simulink model "ble"  (R2020a)
settings: Solver=FixedStepAuto  StartTime=0.0  StopTime=10.0  RelTol=1e-3
undefined symbols (not defined in the file): B3, B7, BLE_Receive, BLE_Send, data, F0, untitled
libraries: androidcommunicationlib x2, androiduilib x2
settings Model: Creator=luisi  LastModifiedBy=luisi
settings OptimizationCC: EnhancedBackFolding=on  PassReuseOutputArgsAs=Individual arguments  ZeroExternalMemoryAtStartup=off  ZeroInternalMemoryAtStartup=off  MaxStackSize=64  OptimizeBlockOrder=speed  DifferentSizesBufferReuse=on  OptimizationCustomize=off  EfficientTunableParamExpr=on
settings DebuggingCC: ParameterTunabilityLossMsg=error
settings HardwareCC: ProdBitPerPointer=32  ProdBitPerSizeT=32  ProdBitPerPtrDiffT=32  ProdLargestAtomicInteger=Long  ProdLargestAtomicFloat=Double  ProdWordSize=32  ProdHWDeviceType=ARM Compatible->ARM Cortex
settings SFSimCC: MATLABDynamicMemAlloc=off
settings RTWCC: SystemTargetFile=ert.tlc  HardwareBoard=Android Device  TemplateMakefile=ert_default_tmf  RTWVerbose=off  Toolchain=Android SDK/NDK Tools
settings CodeAppCC: ForceParamTrailComments=on  IgnoreCustomStorageClasses=off  OperatorAnnotations=on  SimulinkDataObjDesc=on  SFDataObjDesc=on  InsertBlockDesc=on
settings ERTTargetCC: ExtModeMexArgs='192.168.0.149'

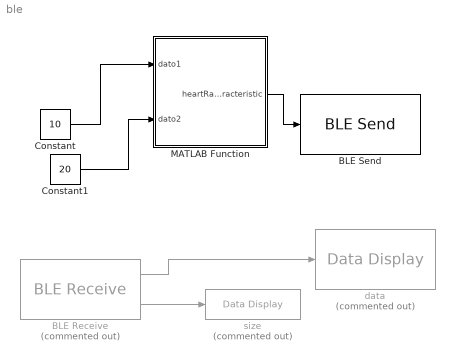
== system ble ==
  BLE Receive : androidcommunicationlib/BLE Receive  Commented=on  DeviceMode=Central (Client)  BluetoothAddress=44:B7:F0:20:80:B3  CharUUID=00002a01-0000-1000-8000-00805f9b34fb  ServiceUUID=00001800-0000-1000-8000-00805f9b34fb  device=RedmiLuisa  character=Generic Access\Appearance  CustomService=off  ServiceName=Heart Rate  CharacteristicName="Heart Rate  Measurement"  CustomServiceUUID=<Enter Service UUID>  CustomCharUUID=<Enter Characteristic UUID>  DataSize=2  SampleTime=0.1  charseruuid=00001801-0000-1000-8000-00805f9b34fb\00002a05-0000-1000-8000-00805f9b34fb  seruuid=00001810-0000-1000-8000-00805f9b34fb  PeripheralService=0000180d-0000-1000-8000-00805f9b34fb  PeripheralCharacteristic=00002a37-0000-1000-8000-00805f9b34fb  chruuid=00002a37-0000-1000-8000-00805f9b34fb  BLEId=untitled/BLE_Receive  Devicename=RedmiLuisa  IsCustomService=0
      settings: SourceProductBaseCode=ANDROID
  BLE Send : androidcommunicationlib/BLE Send  DeviceMode=Peripheral (Server)  BluetoothAddress=44:B7:F0:20:80:B3  CharUUID=00002a05-0000-1000-8000-00805f9b34fb  ServiceUUID=00001801-0000-1000-8000-00805f9b34fb  device=RedmiLuisa  character=Generic Attribute\Service Changed  CustomService=off  ServiceName=Generic Access  CharacteristicName=Appearance  CustomServiceUUID=<Enter Service UUID>  CustomCharUUID=<Enter Characteristic UUID>  charseruuid=00001801-0000-1000-8000-00805f9b34fb\00002a05-0000-1000-8000-00805f9b34fb  seruuid=00001810-0000-1000-8000-00805f9b34fb  chruuid=00002a00-0000-1000-8000-00805f9b34fb  PeripheralService=00001800-0000-1000-8000-00805f9b34fb  PeripheralCharacteristic=00002a01-0000-1000-8000-00805f9b34fb  BLEId=untitled/BLE_Send  Devicename=RedmiLuisa  IsCustomService=0  Size=-1
      settings: SourceProductBaseCode=ANDROID
  Constant : Constant  Value=10
  Constant1 : Constant  Value=20
  MATLAB Function : MATLAB Function  TreatAsAtomicUnit=on
  data : androiduilib/Data Display  Commented=on  DataDisplayId=untitled/data  Format=Float  Precision=1  SimulateUsing=Code generation  blockPlatform=Android
      settings: SourceProductBaseCode=ANDROID
  size : androiduilib/Data Display  Commented=on  DataDisplayId=untitled/size  Format=Float  Precision=1  SimulateUsing=Code generation  blockPlatform=Android
      settings: SourceProductBaseCode=ANDROID
  wires:
  MATLAB Function/1(heartRateCharacteristic) -> BLE Send/1
  Constant/1 -> MATLAB Function/1(dato1)
  BLE Receive/2 -> size/1
  BLE Receive/1 -> data/1
  Constant1/1 -> MATLAB Function/2(dato2)

== matlab function ble/MATLAB Function ==
  data: dato1 input; heartRateCharacteristic output; dato2 input
function heartRateCharacteristic = Convert(dato1, dato2)
flag = uint8(25);
heartRateCharacteristic = zeros(5,1,'uint8');
heartRateCharacteristic(1)= flag;
[lower, upper] = getBytes(dato1);
heartRateCharacteristic(2) = lower;
heartRateCharacteristic(3) = upper;
[lower, upper] = getBytes(dato2);
heartRateCharacteristic(4) = lower;
heartRateCharacteristic(5) = upper;
end

function [lower,upper] = getBytes(parameter)
h = dec2bin(parameter,16);
lower = bin2dec(h(9:16));
upper= bin2dec(h(1:8));
end
